simulink model "stepper_model_Harness1"  (R2018b)
settings: Solver=VariableStepAuto  StartTime=0.0  StopTime=12  FixedStep=0.0001  MaxStep=0.01  RelTol=1e-3  EnableMultiTasking=on
undefined symbols (not defined in the file): sigbuilder_block
settings Model: Creator=Kacper  LastModifiedBy=Kacper
settings DataIOCC: LimitDataPoints=on
settings OptimizationCC: LifeSpan=inf
settings DebuggingCC: AllowSymbolicDim=off  SFUnexpectedBacktrackingDiag=warning  SFNoUnconditionalDefaultTransitionDiag=warning  SFExecutionAtInitializationDiag=none
settings ModelReferenceCC: PropagateSignalLabelsOutOfModel=off
settings SFSimCC: SimUseLocalCustomCode=off
settings RTWCC: RTWUseLocalCustomCode=off
settings CodeAppCC: StateflowObjectComments=on
settings GRTTargetCC: TargetLangStandard=C89/C90 (ANSI)
settings ConfigComp: CovMetricSettings=dw  CovHtmlReporting=on  CovSaveCumulativeToWorkspaceVar=on  CovSaveSingleToWorkspaceVar=on  CovExternalEMLEnable=off

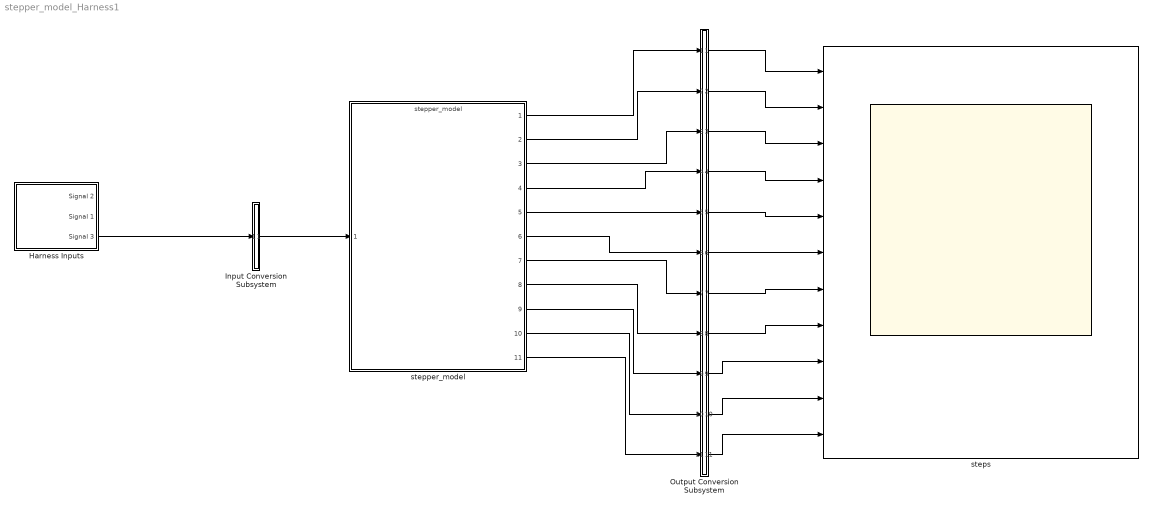
== system stepper_model_Harness1 ==
  Harness Inputs : Subsystem  Tag=STV Subsys  LoadFcn=sigbuilder_block('load',[96 270 822 399.75 ]);  StartFcn=sigbuilder_block('start');  StopFcn=sigbuilder_block('stop');  ClipboardFcn=sigbuilder_block('clipboard');  mask(Sigbuilder block){tuvar=[0:10]}
      mask init:
      | if ~strcmp(get_param(bdroot(gcb),'SimulationStatus'),'stopped'),tuvar = sigbuilder_block('maskInit'); end
      settings: CopyFcn=sigbuilder_block('copy');  DeleteFcn=sigbuilder_block('delete');  ModelCloseFcn=sigbuilder_block('modelClose');  PreSaveFcn=sigbuilder_block('preSave');  PauseFcn=sigbuilder_block('pause');  ContinueFcn=sigbuilder_block('continue');  NameChangeFcn=sigbuilder_block('namechange');  OpenFcn=sigbuilder_block('open',[96 270 822 399.75 ]);  CloseFcn=sigbuilder_block('close');
      mask Display: plot(0, 0, 100, 100,[2, 2, 32, 32, 2], [68, 8, 8, 68, 68],[32, 2], [38, 38], [32, 19, 2],[53, 60, 44], [32, 17, 17, 2],[16, 16, 31, 31]);txt = getActiveGroup(gcbh);text(2, 100, txt,'verticalAlignment', 'top');
  Input Conversion Subsystem : Subsystem  Tag=__SLT_ICS__  Description=|
      | Signal spec.
      | and routing
      settings: AttributesFormatString=%<Description>
  Output Conversion Subsystem : Subsystem  Tag=__SLT_OCS__  Description=|
      | Signal spec.
      | and routing
      settings: AttributesFormatString=%<Description>
  stepper_model : ModelReference  ModelNameDialog=stepper_model  SimulationMode=Normal  ModelReferenceVersion=1.61
  steps : Scope
  wires:
  Output Conversion Subsystem/1(Outport_1) -> steps/1
  Output Conversion Subsystem/2(Outport_2) -> steps/2
  Output Conversion Subsystem/3(Outport_3) -> steps/3
  Output Conversion Subsystem/4(Outport_4) -> steps/4
  Output Conversion Subsystem/5(Outport_5) -> steps/5
  Output Conversion Subsystem/6(Outport_6) -> steps/6
  Output Conversion Subsystem/7(Outport_7) -> steps/7
  Output Conversion Subsystem/8(Outport_8) -> steps/8
  Output Conversion Subsystem/9(Outport_9) -> steps/9
  Output Conversion Subsystem/10(Outport_10) -> steps/10
  Output Conversion Subsystem/11(Outport_11) -> steps/11
  Input Conversion Subsystem/1(Outport_1) -> stepper_model/1
  stepper_model/1 -> Output Conversion Subsystem/1(Inport_1)
  stepper_model/2 -> Output Conversion Subsystem/2(Inport_2)
  stepper_model/3 -> Output Conversion Subsystem/3(Inport_3)
  stepper_model/4 -> Output Conversion Subsystem/4(Inport_4)
  stepper_model/5 -> Output Conversion Subsystem/5(Inport_5)
  stepper_model/6 -> Output Conversion Subsystem/6(Inport_6)
  stepper_model/7 -> Output Conversion Subsystem/7(Inport_7)
  stepper_model/8 -> Output Conversion Subsystem/8(Inport_8)
  stepper_model/9 -> Output Conversion Subsystem/9(Inport_9)
  stepper_model/10 -> Output Conversion Subsystem/10(Inport_10)
  stepper_model/11 -> Output Conversion Subsystem/11(Inport_11)
  Harness Inputs/3(Signal 3) -> Input Conversion Subsystem/1(Inport_1)

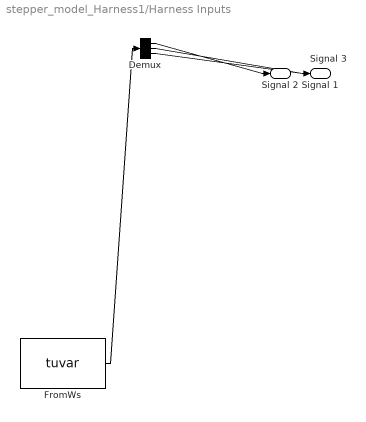
== system stepper_model_Harness1/Harness Inputs ==
  Demux : Demux  Tag=STV Demux  Outputs=3
  FromWs : FromWorkspace  Tag=STV FromWs  VariableName=tuvar  SampleTime=0
      SigBuilderData=|
      | dataSet.timeRange = [0 12]
      | dataSet.name = 'Group 1'
      | sbobj.Name = 'Signal Builder'
      | sbobj.Groups.Name = 'Group 1'
      | sbobj.Groups.Signals(1).Name = 'Signal 2'
      | sbobj.Groups.Signals(1).XData = [0 12]
      | sbobj.Groups.Signals(1).YData = [0.5 0.5]
      | sbobj.Groups.Signals(2).Name = 'Signal 1'
      | sbobj.Groups.Signals(2).XData = [0 4 4 12]
      | sbobj.Groups.Signals(2).YData = [0 0 0.5 0.5]
      | sbobj.Groups.Signals(3).Name = 'Signal 3'
      | sbobj.Groups.Signals(3).XData = [0 0.6 0.6 6 6 12]
      | sbobj.Groups.Signals(3).YData = [0 0 0.3 0.3 0 0]
      | sbobj.Groups.TimeRange = [0 12]
  Signal 2 : Outport  Tag=STV Outport
  Signal 1 : Outport  Tag=STV Outport  Port=2
  Signal 3 : Outport  Tag=STV Outport  Port=3
  wires:
  FromWs/1 -> Demux/1
  Demux/1 -> Signal 2/1
  Demux/2 -> Signal 1/1
  Demux/3 -> Signal 3/1

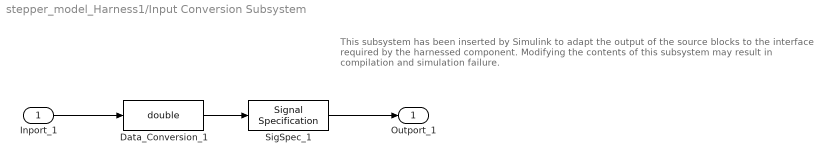
== system stepper_model_Harness1/Input Conversion Subsystem ==
  note: This subsystem has been inserted by Simulink to adapt the output of the source blocks to the interface required by the harnessed component.
      |  Modifying the contents of this subsystem may result in compilation and simulation failure.
  Inport_1 : Inport
  Data_Conversion_1 : DataTypeConversion  OutDataTypeStr=double  SaturateOnIntegerOverflow=on  RndMeth=Zero
  SigSpec_1 : SignalSpecification  OutDataTypeStr=double  Dimensions=[1]  SampleTime=[0, 0]
  Outport_1 : Outport
  wires:
  SigSpec_1/1 -> Outport_1/1
  Data_Conversion_1/1 -> SigSpec_1/1
  Inport_1/1 -> Data_Conversion_1/1

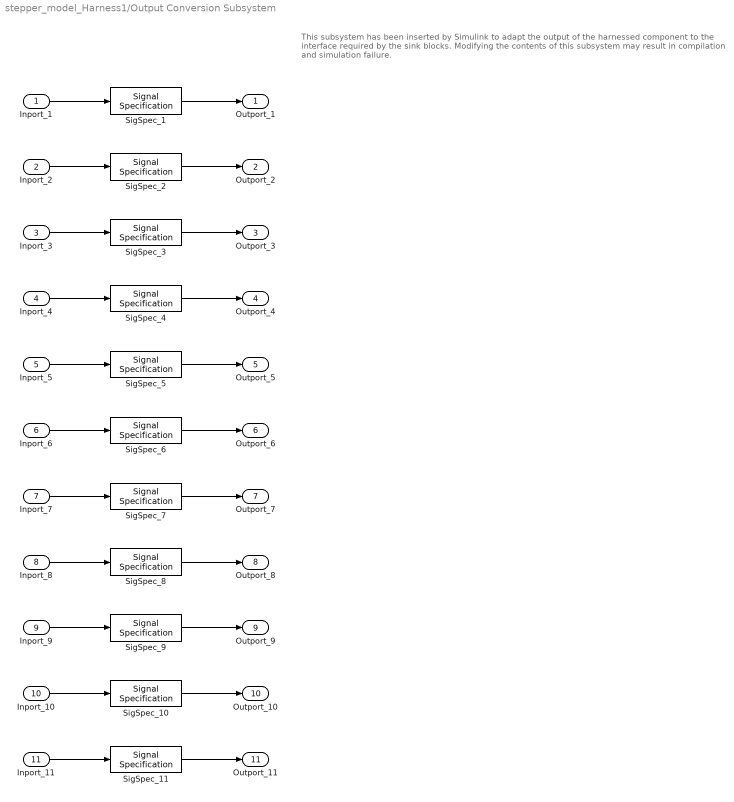
== system stepper_model_Harness1/Output Conversion Subsystem ==
  note: This subsystem has been inserted by Simulink to adapt the output of the harnessed component to the interface required by the sink blocks.
      |  Modifying the contents of this subsystem may result in compilation and simulation failure.
  Inport_1 : Inport
  Inport_2 : Inport  Port=2
  Inport_3 : Inport  Port=3
  Inport_4 : Inport  Port=4
  Inport_5 : Inport  Port=5
  Inport_6 : Inport  Port=6
  Inport_7 : Inport  Port=7
  Inport_8 : Inport  Port=8
  Inport_9 : Inport  Port=9
  Inport_10 : Inport  Port=10
  Inport_11 : Inport  Port=11
  SigSpec_1 : SignalSpecification  OutDataTypeStr=double  Unit=deg  Dimensions=[1]
  SigSpec_{2..11} (10 alike) : SignalSpecification  OutDataTypeStr=double  Unit=1  Dimensions=[1]
  Outport_1 : Outport
  Outport_2 : Outport  Port=2
  Outport_3 : Outport  Port=3
  Outport_4 : Outport  Port=4
  Outport_5 : Outport  Port=5
  Outport_6 : Outport  Port=6
  Outport_7 : Outport  Port=7
  Outport_8 : Outport  Port=8
  Outport_9 : Outport  Port=9
  Outport_10 : Outport  Port=10
  Outport_11 : Outport  Port=11
  wires:
  Inport_1/1 -> SigSpec_1/1
  SigSpec_1/1 -> Outport_1/1
  Inport_2/1 -> SigSpec_2/1
  SigSpec_2/1 -> Outport_2/1
  Inport_3/1 -> SigSpec_3/1
  SigSpec_3/1 -> Outport_3/1
  Inport_4/1 -> SigSpec_4/1
  SigSpec_4/1 -> Outport_4/1
  Inport_5/1 -> SigSpec_5/1
  SigSpec_5/1 -> Outport_5/1
  Inport_6/1 -> SigSpec_6/1
  SigSpec_6/1 -> Outport_6/1
  Inport_7/1 -> SigSpec_7/1
  SigSpec_7/1 -> Outport_7/1
  Inport_8/1 -> SigSpec_8/1
  SigSpec_8/1 -> Outport_8/1
  Inport_9/1 -> SigSpec_9/1
  SigSpec_9/1 -> Outport_9/1
  Inport_10/1 -> SigSpec_10/1
  SigSpec_10/1 -> Outport_10/1
  Inport_11/1 -> SigSpec_11/1
  SigSpec_11/1 -> Outport_11/1
